simulink model "VIPR557LTStEnCtrl"  (R2024b)
settings: Solver=FixedStepDiscrete  StartTime=0.0  StopTime=10.0  FixedStep=0.01  RelTol=1e-3
undefined symbols (not defined in the file or in its folder): data, KeSMSw4SSecRwLtStLgrstUpwdDnwdOpenPos1_Val, PassStBkReclnEn_Clear, PassStBkReclnEn_Set, PassStFwdBkwdEn_Clear, PassStFwdBkwdEn_Set, SecRwRtStBkReclnEn_Clear, SecRwRtStBkReclnEn_Set, SecRwRtStFwdBkwdEn_Clear, SecRwRtStFwdBkwdEn_Set, SecRwRtStLgrstInwdOtwdEn_Clear, SecRwRtStLgrstInwdOtwdEn_Set, SecRwRtStLgrstUpwdDnwdEn_Clear, SecRwRtStLgrstUpwdDnwdEn_Set, ThdRwLtStBkReclnEn_Clear, ThdRwLtStBkReclnEn_Set, ThdRwLtStFwdBkwdEn_Clear, ThdRwLtStFwdBkwdEn_Set, ThdRwRtStBkReclnEn_Clear, ThdRwRtStBkReclnEn_Set, ThdRwRtStFwdBkwdEn_Clear, ThdRwRtStFwdBkwdEn_Set
libraries: simulink x1
settings Model: Creator=sn2xws  LastModifiedBy=sn55gm
settings Model: ModifiedHistory=|
  | 2024.7.3 V3.0.0 557模式流程V1.9
  | 2024.10.28 V3.0.1 6s不动三左
  | 2024.11.29 V3.0.2 7s信号未连接
  | 2024.12.2 V3.0.3 SecRwLtStLgrstOtwdInwdStgDone错误使用SecRwLtStLgrstUpwdDnwdStgDone信号
  | 2024.12.11 V3.0.4 CR960452
settings SolverCC: AlgebraicLoopSolver=TrustRegion
settings DataIOCC: SaveFormat=StructureWithTime  ReturnWorkspaceOutputs=off
settings OptimizationCC: DefaultParameterBehavior=Inlined  EnhancedBackFolding=on  PassReuseOutputArgsAs=Individual arguments  ZeroExternalMemoryAtStartup=off  ZeroInternalMemoryAtStartup=off  OptimizeBlockOrder=speed  DifferentSizesBufferReuse=on  OptimizationCustomize=off  EfficientTunableParamExpr=on
settings DebuggingCC: ParameterTunabilityLossMsg=error  UnconnectedInputMsg=warning  UnconnectedOutputMsg=warning  UnconnectedLineMsg=warning  ArithmeticOperatorsInVariantConditions=warning
settings ModelReferenceCC: EnableRefExpFcnMdlSchedulingChecks=on
settings SFSimCC: MATLABDynamicMemAlloc=off  CustomCodeUndefinedFunction=UseInterfaceOnly
settings RTWCC: Description=AUTOSAR  SystemTargetFile=autosar.tlc  GenCodeOnly=on  TemplateMakefile=ert_default_tmf  GenerateReport=on  IncludeHyperlinkInReport=on  LaunchReport=on  DataTypeReplacement=CDataTypesFixedWidth  GenerateTraceInfo=on  GenerateTraceReport=on  GenerateTraceReportSl=on  GenerateTraceReportSf=on  GenerateTraceReportEml=on  GPUComputeCapability=3.5
settings CodeAppCC: ForceParamTrailComments=on  IgnoreCustomStorageClasses=off  OperatorAnnotations=on  SimulinkDataObjDesc=on  SFDataObjDesc=on  InsertBlockDesc=on
settings STFCustomTargetCC: TargetLangStandard=C99 (ISO)  MultiwordLength=256  ParMdlRefBuildCompliant=on  CompOptLevelCompliant=on  IncludeMdlTerminateFcn=off  CombineOutputUpdateFcns=on  SuppressErrorStatus=on  ERTCustomFileBanners=on  SupportNonFinite=off  SupportComplex=off  SupportContinuousTime=off  SupportNonInlinedSFcns=off  RemoveResetFunc=on  MATLABClassNameForMDSCustomization=Simulink.SoftwareTarget.ERTCustomization  AutosarCompliant=on  UseToolchainInfoCompliant=on  LookupTableObjectStructAxisOrder=2,1,3,4,...  LUTObjectStructOrderEvenSpacing=Size,Table,Breakpoints  SystemTargetFile=autosar.tlc
settings ERTTargetCC: TargetLangStandard=C99 (ISO)  ConcurrentExecutionCompliant=off  IncludeMdlTerminateFcn=off  SuppressErrorStatus=on  SupportNonFinite=off  SupportComplex=off  ModelStepFunctionPrototypeControlCompliant=off  CPPClassGenCompliant=off  AutosarCompliant=on  LookupTableObjectStructAxisOrder=2,1,3,4,...  LUTObjectStructOrderEvenSpacing=Size,Table,Breakpoints  ERTCustomFileTemplate=example_file_process.tlc  ERTFilePackagingFormat=Compact  BooleanTrueId=TRUE  BooleanFalseId=FALSE  DynamicArrayContainerType=coder::array

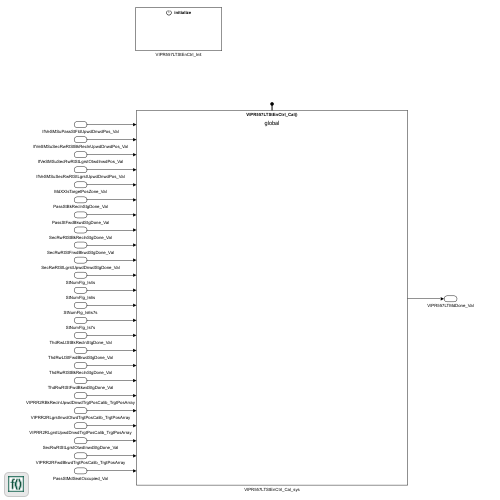
[thumbnail: Simulink's stored preview of the top-level diagram]
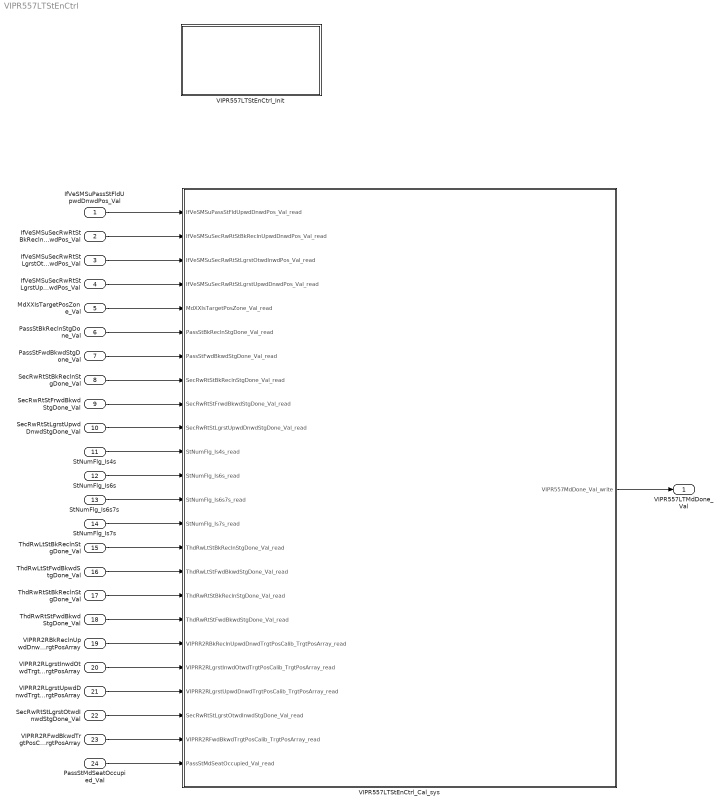
== system VIPR557LTStEnCtrl ==
  IfVeSMSuPassStFldUpwdDnwdPos_Val : Inport  OutDataTypeStr=uint16  PortDimensions=1
  IfVeSMSuSecRwRtStBkReclnUpwdDnwdPos_Val : Inport  Port=2  OutDataTypeStr=uint16  PortDimensions=1
  IfVeSMSuSecRwRtStLgrstOtwdInwdPos_Val : Inport  Port=3  OutDataTypeStr=uint16  PortDimensions=1
  IfVeSMSuSecRwRtStLgrstUpwdDnwdPos_Val : Inport  Port=4  OutDataTypeStr=uint16  PortDimensions=1
  MdXXIsTargetPosZone_Val : Inport  Port=5  OutDataTypeStr=uint32  PortDimensions=1
  PassStBkReclnStgDone_Val : Inport  Port=6  OutDataTypeStr=boolean  PortDimensions=1
  PassStFwdBkwdStgDone_Val : Inport  Port=7  OutDataTypeStr=boolean  PortDimensions=1
  SecRwRtStBkReclnStgDone_Val : Inport  Port=8  OutDataTypeStr=boolean  PortDimensions=1
  SecRwRtStFrwdBkwdStgDone_Val : Inport  Port=9  OutDataTypeStr=boolean  PortDimensions=1
  SecRwRtStLgrstUpwdDnwdStgDone_Val : Inport  Port=10  OutDataTypeStr=boolean  PortDimensions=1
  StNumFlg_Is4s : Inport  Port=11  OutDataTypeStr=boolean  PortDimensions=1
  StNumFlg_Is6s : Inport  Port=12  OutDataTypeStr=boolean  PortDimensions=1
  StNumFlg_Is6s7s : Inport  Port=13  OutDataTypeStr=boolean  PortDimensions=1
  StNumFlg_Is7s : Inport  Port=14  OutDataTypeStr=boolean  PortDimensions=1
  ThdRwLtStBkReclnStgDone_Val : Inport  Port=15  OutDataTypeStr=boolean  PortDimensions=1
  ThdRwLtStFwdBkwdStgDone_Val : Inport  Port=16  OutDataTypeStr=boolean  PortDimensions=1
  ThdRwRtStBkReclnStgDone_Val : Inport  Port=17  OutDataTypeStr=boolean  PortDimensions=1
  ThdRwRtStFwdBkwdStgDone_Val : Inport  Port=18  OutDataTypeStr=boolean  PortDimensions=1
  VIPRR2RBkReclnUpwdDnwdTrgtPosCalib_TrgtPosArray : Inport  Description=|  Port=19  OutDataTypeStr=uint16  PortDimensions=3
      | 0:Pos
      | 1:Max
      | 2:Min
  VIPRR2RLgrstInwdOtwdTrgtPosCalib_TrgtPosArray : Inport  Description=|  Port=20  OutDataTypeStr=uint16  PortDimensions=3
      | 0:Pos
      | 1:Max
      | 2:Min
  VIPRR2RLgrstUpwdDnwdTrgtPosCalib_TrgtPosArray : Inport  Description=|  Port=21  OutDataTypeStr=uint16  PortDimensions=3
      | 0:Pos
      | 1:Max
      | 2:Min
  SecRwRtStLgrstOtwdInwdStgDone_Val : Inport  Port=22  OutDataTypeStr=boolean  PortDimensions=1
  VIPRR2RFwdBkwdTrgtPosCalib_TrgtPosArray : Inport  Description=|  Port=23  OutDataTypeStr=uint16  PortDimensions=3
      | 0:Pos
      | 1:Max
      | 2:Min
  PassStMdSeatOccupied_Val : Inport  Port=24  OutDataTypeStr=boolean  PortDimensions=1
  VIPR557LTStEnCtrl_Cal_sys : Subsystem
  VIPR557LTStEnCtrl_Init : Subsystem
  VIPR557LTMdDone_Val : Outport  OutDataTypeStr=uint8  PortDimensions=1  VectorParamsAs1DForOutWhenUnconnected=off
  wires:
  IfVeSMSuPassStFldUpwdDnwdPos_Val/1 -> VIPR557LTStEnCtrl_Cal_sys/1(IfVeSMSuPassStFldUpwdDnwdPos_Val_read)
  IfVeSMSuSecRwRtStBkReclnUpwdDnwdPos_Val/1 -> VIPR557LTStEnCtrl_Cal_sys/2(IfVeSMSuSecRwRtStBkReclnUpwdDnwdPos_Val_read)
  IfVeSMSuSecRwRtStLgrstOtwdInwdPos_Val/1 -> VIPR557LTStEnCtrl_Cal_sys/3(IfVeSMSuSecRwRtStLgrstOtwdInwdPos_Val_read)
  IfVeSMSuSecRwRtStLgrstUpwdDnwdPos_Val/1 -> VIPR557LTStEnCtrl_Cal_sys/4(IfVeSMSuSecRwRtStLgrstUpwdDnwdPos_Val_read)
  MdXXIsTargetPosZone_Val/1 -> VIPR557LTStEnCtrl_Cal_sys/5(MdXXIsTargetPosZone_Val_read)
  PassStBkReclnStgDone_Val/1 -> VIPR557LTStEnCtrl_Cal_sys/6(PassStBkReclnStgDone_Val_read)
  PassStFwdBkwdStgDone_Val/1 -> VIPR557LTStEnCtrl_Cal_sys/7(PassStFwdBkwdStgDone_Val_read)
  SecRwRtStBkReclnStgDone_Val/1 -> VIPR557LTStEnCtrl_Cal_sys/8(SecRwRtStBkReclnStgDone_Val_read)
  SecRwRtStFrwdBkwdStgDone_Val/1 -> VIPR557LTStEnCtrl_Cal_sys/9(SecRwRtStFrwdBkwdStgDone_Val_read)
  SecRwRtStLgrstUpwdDnwdStgDone_Val/1 -> VIPR557LTStEnCtrl_Cal_sys/10(SecRwRtStLgrstUpwdDnwdStgDone_Val_read)
  StNumFlg_Is4s/1 -> VIPR557LTStEnCtrl_Cal_sys/11(StNumFlg_Is4s_read)
  StNumFlg_Is6s/1 -> VIPR557LTStEnCtrl_Cal_sys/12(StNumFlg_Is6s_read)
  StNumFlg_Is6s7s/1 -> VIPR557LTStEnCtrl_Cal_sys/13(StNumFlg_Is6s7s_read)
  StNumFlg_Is7s/1 -> VIPR557LTStEnCtrl_Cal_sys/14(StNumFlg_Is7s_read)
  ThdRwLtStBkReclnStgDone_Val/1 -> VIPR557LTStEnCtrl_Cal_sys/15(ThdRwLtStBkReclnStgDone_Val_read)
  ThdRwLtStFwdBkwdStgDone_Val/1 -> VIPR557LTStEnCtrl_Cal_sys/16(ThdRwLtStFwdBkwdStgDone_Val_read)
  ThdRwRtStBkReclnStgDone_Val/1 -> VIPR557LTStEnCtrl_Cal_sys/17(ThdRwRtStBkReclnStgDone_Val_read)
  ThdRwRtStFwdBkwdStgDone_Val/1 -> VIPR557LTStEnCtrl_Cal_sys/18(ThdRwRtStFwdBkwdStgDone_Val_read)
  VIPRR2RBkReclnUpwdDnwdTrgtPosCalib_TrgtPosArray/1 -> VIPR557LTStEnCtrl_Cal_sys/19(VIPRR2RBkReclnUpwdDnwdTrgtPosCalib_TrgtPosArray_read)
  VIPRR2RLgrstInwdOtwdTrgtPosCalib_TrgtPosArray/1 -> VIPR557LTStEnCtrl_Cal_sys/20(VIPRR2RLgrstInwdOtwdTrgtPosCalib_TrgtPosArray_read)
  VIPRR2RLgrstUpwdDnwdTrgtPosCalib_TrgtPosArray/1 -> VIPR557LTStEnCtrl_Cal_sys/21(VIPRR2RLgrstUpwdDnwdTrgtPosCalib_TrgtPosArray_read)
  VIPR557LTStEnCtrl_Cal_sys/1(VIPR557MdDone_Val_write) -> VIPR557LTMdDone_Val/1
  SecRwRtStLgrstOtwdInwdStgDone_Val/1 -> VIPR557LTStEnCtrl_Cal_sys/22(SecRwRtStLgrstOtwdInwdStgDone_Val_read)
  VIPRR2RFwdBkwdTrgtPosCalib_TrgtPosArray/1 -> VIPR557LTStEnCtrl_Cal_sys/23(VIPRR2RFwdBkwdTrgtPosCalib_TrgtPosArray_read)
  PassStMdSeatOccupied_Val/1 -> VIPR557LTStEnCtrl_Cal_sys/24(PassStMdSeatOccupied_Val_read)

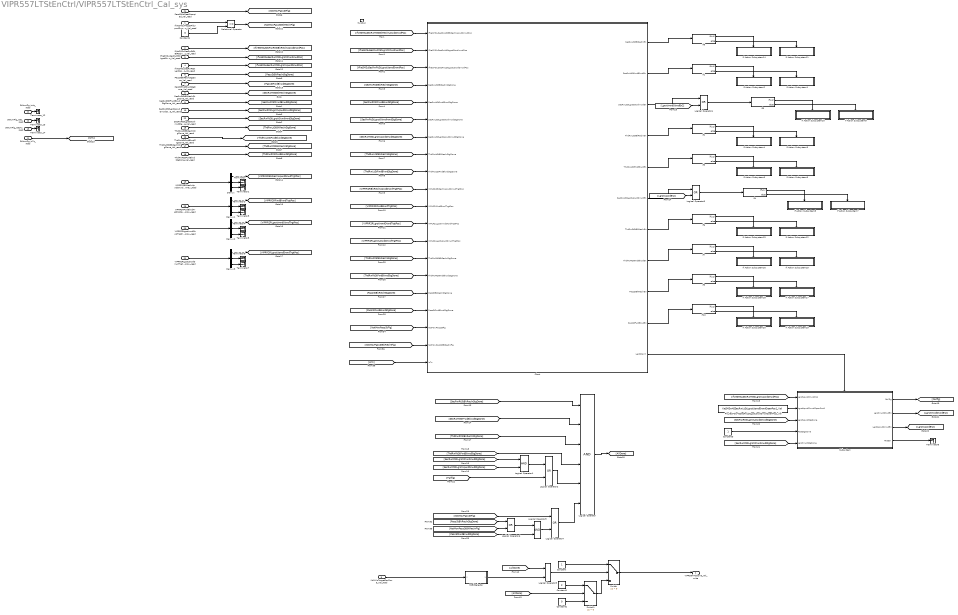
== system VIPR557LTStEnCtrl/VIPR557LTStEnCtrl_Cal_sys ==
  IfVeSMSuPassStFldUpwdDnwdPos_Val_read : Inport
  IfVeSMSuSecRwRtStBkReclnUpwdDnwdPos_Val_read : Inport  Port=2
  IfVeSMSuSecRwRtStLgrstOtwdInwdPos_Val_read : Inport  Port=3
  IfVeSMSuSecRwRtStLgrstUpwdDnwdPos_Val_read : Inport  Port=4
  MdXXIsTargetPosZone_Val_read : Inport  Port=5
  PassStBkReclnStgDone_Val_read : Inport  Port=6
  PassStFwdBkwdStgDone_Val_read : Inport  Port=7
  SecRwRtStBkReclnStgDone_Val_read : Inport  Port=8
  SecRwRtStFrwdBkwdStgDone_Val_read : Inport  Port=9
  SecRwRtStLgrstUpwdDnwdStgDone_Val_read : Inport  Port=10
  StNumFlg_Is4s_read : Inport  Port=11
  StNumFlg_Is6s_read : Inport  Port=12
  StNumFlg_Is6s7s_read : Inport  Port=13
  StNumFlg_Is7s_read : Inport  Port=14
  ThdRwLtStBkReclnStgDone_Val_read : Inport  Port=15
  ThdRwLtStFwdBkwdStgDone_Val_read : Inport  Port=16
  ThdRwRtStBkReclnStgDone_Val_read : Inport  Port=17
  ThdRwRtStFwdBkwdStgDone_Val_read : Inport  Port=18
  VIPRR2RBkReclnUpwdDnwdTrgtPosCalib_TrgtPosArray_read : Inport  Port=19
  VIPRR2RLgrstInwdOtwdTrgtPosCalib_TrgtPosArray_read : Inport  Port=20
  VIPRR2RLgrstUpwdDnwdTrgtPosCalib_TrgtPosArray_read : Inport  Port=21
  SecRwRtStLgrstOtwdInwdStgDone_Val_read : Inport  Port=22
  VIPRR2RFwdBkwdTrgtPosCalib_TrgtPosArray_read : Inport  Port=23
  PassStMdSeatOccupied_Val_read : Inport  Port=24
  function : TriggerPort  TriggerType=function-call  IsSimulinkFunction=on  FunctionName=VIPR557LTStEnCtrl_Cal  VariantControl=(inherit)
  32BitSelector : Subsystem  mask(32 Bit Selector){BitNum=11}
      mask prompts: BitNum "Select Bit Number"
      mask help: Allows selection of a particular bit (0-31) out of a packed word up to 32 bits long. Output will be true if the bit number selected via the mask parameter is equal to one.
      mask TypeOptions BitNum: 0 | 1 | 2 | 3 | 4 | 5 | 6 | 7 | 8 | 9 | 10 | 11 | 12 | 13 | 14 | 15 | 16 | 17 | 18 | 19 | 20 | 21 | 22 | 23 | 24 | 25 | 26 | 27 | 28 | 29 | 30 | 31
      mask Display:
      | text(0.5, 0.8,'BIT','horizontalAlignment','center')
      | text(0.5, 0.5,'SELECTOR','horizontalAlignment','center')
      | text(0.5, 0.2,['-- Bit ',char(get_param(gcb,'BitNum')),' --'],'horizontalAlignment','center')
  Chart : Stateflow chart  TreatAsAtomicUnit=on
  Constant : Constant  OutDataTypeStr=uint8
  Constant1 : Constant  Value=2  OutDataTypeStr=uint8
  Constant2 : Constant  Value=0  OutDataTypeStr=uint8
  Constant3 : Constant  OutDataTypeStr=boolean
  Constant4 : Constant  Value=0  OutDataTypeStr=uint16
  Demux{,1..3} (4 alike) : Demux  Outputs=3
  If Action Subsystem1 : Subsystem  TreatAsAtomicUnit=on
  If Action Subsystem10 : Subsystem  TreatAsAtomicUnit=on
  If Action Subsystem11 : Subsystem  TreatAsAtomicUnit=on
  If Action Subsystem12 : Subsystem  TreatAsAtomicUnit=on
  If Action Subsystem13 : Subsystem  TreatAsAtomicUnit=on
  If Action Subsystem14 : Subsystem  TreatAsAtomicUnit=on
  If Action Subsystem15 : Subsystem  TreatAsAtomicUnit=on
  If Action Subsystem16 : Subsystem  TreatAsAtomicUnit=on
  If Action Subsystem17 : Subsystem  TreatAsAtomicUnit=on
  If Action Subsystem18 : Subsystem  TreatAsAtomicUnit=on
  If Action Subsystem19 : Subsystem  TreatAsAtomicUnit=on
  If Action Subsystem2 : Subsystem  TreatAsAtomicUnit=on
  If Action Subsystem20 : Subsystem  TreatAsAtomicUnit=on
  If Action Subsystem3 : Subsystem  TreatAsAtomicUnit=on
  If Action Subsystem4 : Subsystem  TreatAsAtomicUnit=on
  If Action Subsystem5 : Subsystem  TreatAsAtomicUnit=on
  If Action Subsystem6 : Subsystem  TreatAsAtomicUnit=on
  If Action Subsystem7 : Subsystem  TreatAsAtomicUnit=on
  If Action Subsystem8 : Subsystem  TreatAsAtomicUnit=on
  If Action Subsystem9 : Subsystem  TreatAsAtomicUnit=on
  If{1..10} (10 alike) : If  IfExpression=u1
  Logical Operator : Logic  Inputs=6  AllPortsSameDT=off  OutDataTypeStr=boolean
  Logical Operator1 : Logic  AllPortsSameDT=off  OutDataTypeStr=boolean
  Logical Operator{2..4,6..7} (5 alike) : Logic  Operator=OR  AllPortsSameDT=off  OutDataTypeStr=boolean
  Logical Operator5 : Logic  AllPortsSameDT=off  OutDataTypeStr=boolean
  Logical Operator9 : Logic  AllPortsSameDT=off  OutDataTypeStr=boolean
  PA_KeSMSw4SSecRwLtStLgrstUpwdDnwdOpenPos1_Val : Constant  Value=KeSMSw4SSecRwLtStLgrstUpwdDnwdOpenPos1_Val
  Relational Operator : RelationalOperator  Operator=<=  OutDataTypeStr=boolean  RndMeth=Simplest  InputSameDT=off
  Subsystem : Subsystem
  Switch : Switch  Criteria=u2 > Threshold  SaturateOnIntegerOverflow=off  InputSameDT=off
  Switch1 : Switch  Criteria=u2 > Threshold  SaturateOnIntegerOverflow=off  InputSameDT=off
  Terminator{,1..8} (9 alike) : Terminator
  Terminator_12 : Terminator
  Terminator_13 : Terminator
  Terminator_14 : Terminator
  VIPR557MdDone_Val_write : Outport  VectorParamsAs1DForOutWhenUnconnected=off
      settings: EnsureOutportIsVirtual=on
  wires:
  StNumFlg_Is4s_read/1 -> Terminator_12/1
  StNumFlg_Is6s_read/1 -> Terminator_13/1
  StNumFlg_Is6s7s_read/1 -> Terminator_14/1
  StNumFlg_Is7s_read/1 -> [Is7s]
  ThdRwLtStBkReclnStgDone_Val_read/1 -> [ThdRwLtStBkReclnStgDone]
  SecRwRtStFrwdBkwdStgDone_Val_read/1 -> [SecRwRtStFrwdBkwdStgDone]
  SecRwRtStLgrstUpwdDnwdStgDone_Val_read/1 -> [SecRwRtStLgrstUpwdDnwdStgDone]
  SecRwRtStBkReclnStgDone_Val_read/1 -> [SecRwRtStBkReclnStgDone]
  ThdRwLtStFwdBkwdStgDone_Val_read/1 -> [ThdRwLtStFwdBkwdStgDone]
  SecRwRtStLgrstOtwdInwdStgDone_Val_read/1 -> [SecRwRtStLgrstOtwdInwdStgDone]
  IfVeSMSuSecRwRtStBkReclnUpwdDnwdPos_Val_read/1 -> [IfVeSMSuSecRwRtStBkReclnUpwdDnwdPos]
  IfVeSMSuSecRwRtStLgrstOtwdInwdPos_Val_read/1 -> [IfVeSMSuSecRwRtStLgrstOtwdInwdPos]
  IfVeSMSuSecRwRtStLgrstUpwdDnwdPos_Val_read/1 -> [IfVeSMSuSecRwRtStLgrstUpwdDnwdPos]
  ThdRwRtStBkReclnStgDone_Val_read/1 -> [ThdRwRtStBkReclnStgDone]
  ThdRwRtStFwdBkwdStgDone_Val_read/1 -> [ThdRwRtStFwdBkwdStgDone]
  PassStBkReclnStgDone_Val_read/1 -> [PassStBkReclnStgDone]
  PassStFwdBkwdStgDone_Val_read/1 -> [PassStFwdBkwdStgDone]
  Demux2/1 -> [VIPRR2RLgrstInwdOtwdTrgtPos]
  VIPRR2RBkReclnUpwdDnwdTrgtPosCalib_TrgtPosArray_read/1 -> Demux/1
  VIPRR2RFwdBkwdTrgtPosCalib_TrgtPosArray_read/1 -> Demux1/1
  VIPRR2RLgrstUpwdDnwdTrgtPosCalib_TrgtPosArray_read/1 -> Demux3/1
  Demux3/1 -> [VIPRR2RLgrstUpwdDnwdTrgtPos]
  Demux3/2 -> Terminator6/1
  Demux1/3 -> Terminator3/1
  Demux/3 -> Terminator1/1
  Demux3/3 -> Terminator7/1
  Demux/1 -> [VIPRR2RBkReclnUpwdDnwdTrgtPos]
  Demux1/1 -> [VIPRR2RFwdBkwdTrgtPos]
  Demux2/2 -> Terminator4/1
  VIPRR2RLgrstInwdOtwdTrgtPosCalib_TrgtPosArray_read/1 -> Demux2/1
  Demux/2 -> Terminator/1
  Demux2/3 -> Terminator5/1
  Demux1/2 -> Terminator2/1
  [IfVeSMSuSecRwRtStLgrstUpwdDnwdPos] -> Chart/3(IfVeSMSuSecRwLtStLgrstUpwdDnwdPos)
  [SecRwRtStFrwdBkwdStgDone] -> Logical Operator/2
  Logical Operator4/1 -> If5/1
  Chart/11(LgrstOpn()) -> Subsystem/Trigger
  [LgrstUpwdEn2] -> Logical Operator3/2
  Chart/3(SecRwLtStLgrstOtwdInwdEn) -> Logical Operator4/1
  Chart/5(ThdRwLtStFwdBkwdEn) -> If3/1
  If5/2 -> If Action Subsystem9/Action
  [SecRwRtStLgrstOtwdInwdStgDone] -> Logical Operator1/1
  If4/1 -> If Action Subsystem8/Action
  Logical Operator2/1 -> Logical Operator/5
  [LgrstInwdOtwdEn2] -> Logical Operator4/2
  Chart/6(SecRwLtStLgrstUpwdDnwdEn) -> Logical Operator3/1
  Chart/4(ThdRwLtStBkReclnEn) -> If2/1
  If1/1 -> If Action Subsystem2/Action
  [IfVeSMSuSecRwRtStLgrstOtwdInwdPos] -> Chart/2(IfVeSMSuSecRwLtStLgrstOtwdInwdPos)
  Subsystem/2(LgrstInwdOtwdEn) -> [LgrstInwdOtwdEn2]
  Logical Operator/1 -> [AllDone]
  [VIPRR2RLgrstInwdOtwdTrgtPos] -> Chart/12(VIPLR2LLgrstInwdOtwdTrgtPos)
  If1/2 -> If Action Subsystem1/Action
  If4/2 -> If Action Subsystem7/Action
  Subsystem/1(Failflg) -> [Failflg]
  [SecRwRtStBkReclnStgDone] -> Logical Operator/1
  Subsystem/4(FtrstEn) -> Terminator8/1
  If8/2 -> If Action Subsystem11/Action
  If2/2 -> If Action Subsystem3/Action
  If3/1 -> If Action Subsystem6/Action
  [SecRwRtStLgrstUpwdDnwdStgDone] -> Subsystem/3(LgrstUpwdStgDone)
  Chart/1(SecRwLtStBkReclnEn) -> If8/1
  [ThdRwRtStFwdBkwdStgDone] -> Logical Operator/4
  [SecRwRtStLgrstUpwdDnwdStgDone] -> Logical Operator1/2
  [Failflg] -> Logical Operator2/2
  [SecRwRtStLgrstOtwdInwdStgDone] -> Subsystem/5(LgrstInwdStgDone)
  [SecRwRtStLgrstUpwdDnwdStgDone] -> Chart/7(SecRwLtStLgrstUpwdDnwdStgDone)
  Subsystem/3(LgrstUpwdDnwdEn) -> [LgrstUpwdEn2]
  Constant3/1 -> Subsystem/4(FtrstStgDone)
  If5/1 -> If Action Subsystem10/Action
  [SecRwRtStFrwdBkwdStgDone] -> Chart/5(SecRwLtStFrwdBkwdStgDone)
  If8/1 -> If Action Subsystem14/Action
  [VIPRR2RLgrstUpwdDnwdTrgtPos] -> Chart/13(VIPLR2LLgrstUpwdDnwdTrgtPos)
  [VIPRR2RFwdBkwdTrgtPos] -> Chart/11(VIPLR2LFwdBkwdTrgtPos)
  Chart/2(SecRwLtStFrwdBkwdEn) -> If1/1
  Logical Operator1/1 -> Logical Operator2/1
  [SecRwRtStBkReclnStgDone] -> Chart/4(SecRwLtStBkReclnStgDone)
  [SecRwRtStLgrstOtwdInwdStgDone] -> Chart/6(SecRwLtStLgrstOtwdInwdStgDone)
  If3/2 -> If Action Subsystem5/Action
  If2/1 -> If Action Subsystem4/Action
  [ThdRwLtStBkReclnStgDone] -> Chart/8(ThdRwLtStBkReclnStgDone)
  PA_KeSMSw4SSecRwLtStLgrstUpwdDnwdOpenPos1_Val/1 -> Subsystem/2(LgrstUpwdDnwdOpenPos1)
  [IfVeSMSuSecRwRtStBkReclnUpwdDnwdPos] -> Chart/1(IfVeSMSuSecRwLtStBkReclnUpwdDnwdPos)
  Logical Operator3/1 -> If4/1
  [VIPRR2RBkReclnUpwdDnwdTrgtPos] -> Chart/10(VIPLR2LBkReclnUpwdDnwdTrgtPos)
  [ThdRwLtStFwdBkwdStgDone] -> Chart/9(ThdRwLtStFwdBkwdStgDone)
  [ThdRwRtStBkReclnStgDone] -> Logical Operator/3
  [IfVeSMSuSecRwRtStLgrstUpwdDnwdPos] -> Subsystem/1(LgrstUpwdDnwdPos)
  [AllDone] -> Logical Operator9/1
  Constant2/1 -> Switch1/3
  32BitSelector/1(y) -> Logical Operator9/2
  Constant1/1 -> Switch1/1
  Switch1/1 -> Switch/3
  Logical Operator9/1 -> Switch/2
  Constant/1 -> Switch/1
  [AllDone] -> Switch1/2
  MdXXIsTargetPosZone_Val_read/1 -> 32BitSelector/1(x)
  Switch/1 -> VIPR557MdDone_Val_write/1
  [PassStBkReclnStgDone] -> Chart/16(PassStBkReclnStgDone)
  Logical Operator7/1 -> Logical Operator/6
  Logical Operator5/1 -> Logical Operator7/2
  IfVeSMSuPassStFldUpwdDnwdPos_Val_read/1 -> Relational Operator/1
  Constant4/1 -> Relational Operator/2
  PassStMdSeatOccupied_Val_read/1 -> [NotMovPassStFlg]
  [NotMovPassStFlg] -> Logical Operator7/1
  Relational Operator/1 -> [NotMovPassStBkReclnFlg]
  [PassStBkReclnStgDone] -> Logical Operator6/1
  [NotMovPassStBkReclnFlg] -> Logical Operator6/2
  Logical Operator6/1 -> Logical Operator5/1
  [PassStFwdBkwdStgDone] -> Logical Operator5/2
  [ThdRwRtStBkReclnStgDone] -> Chart/14(ThdRwRtStBkReclnStgDone)
  [ThdRwRtStFwdBkwdStgDone] -> Chart/15(ThdRwRtStFwdBkwdStgDone)
  [NotMovPassStFlg] -> Chart/18(NotMovPassStFlg)
  [PassStFwdBkwdStgDone] -> Chart/17(PassStFwdBkwdStgDone)
  [NotMovPassStBkReclnFlg] -> Chart/19(NotMovPassStBkReclnFlg)
  If6/2 -> If Action Subsystem12/Action
  If6/1 -> If Action Subsystem13/Action
  Chart/7(ThdRwRtStBkReclnEn) -> If6/1
  Chart/8(ThdRwRtStFwdBkwdEn) -> If7/1
  If7/1 -> If Action Subsystem16/Action
  If7/2 -> If Action Subsystem15/Action
  If9/2 -> If Action Subsystem17/Action
  If9/1 -> If Action Subsystem18/Action
  Chart/9(PassStBkReclnEn) -> If9/1
  Chart/10(PassStFwdBkwdEn) -> If10/1
  If10/1 -> If Action Subsystem20/Action
  If10/2 -> If Action Subsystem19/Action
  [Is7s] -> Chart/20(is7s)

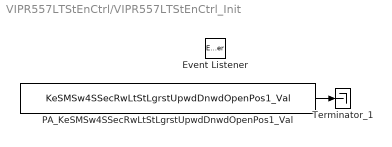
== system VIPR557LTStEnCtrl/VIPR557LTStEnCtrl_Init ==
  Event Listener : EventListener  EventName=reset
  PA_KeSMSw4SSecRwLtStLgrstUpwdDnwdOpenPos1_Val : Constant  Value=KeSMSw4SSecRwLtStLgrstUpwdDnwdOpenPos1_Val
  Terminator_1 : Terminator
  wires:
  PA_KeSMSw4SSecRwLtStLgrstUpwdDnwdOpenPos1_Val/1 -> Terminator_1/1

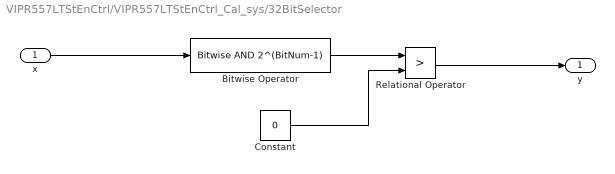
== system VIPR557LTStEnCtrl/VIPR557LTStEnCtrl_Cal_sys/32BitSelector ==
  x : Inport
  Bitwise Operator : simulink/Logic and Bit Operations/Bitwise Operator  logicop=AND  UseBitMask=on  BitMask=2^(BitNum-1)  BitMaskRealWorld=Stored Integer
  Constant : Constant  Value=0  OutDataTypeStr=uint32
  Relational Operator : RelationalOperator  Operator=>  OutDataTypeStr=boolean  RndMeth=Simplest  InputSameDT=off
  y : Outport  VectorParamsAs1DForOutWhenUnconnected=off
  wires:
  Relational Operator/1 -> y/1
  Constant/1 -> Relational Operator/2
  x/1 -> Bitwise Operator/1
  Bitwise Operator/1 -> Relational Operator/1

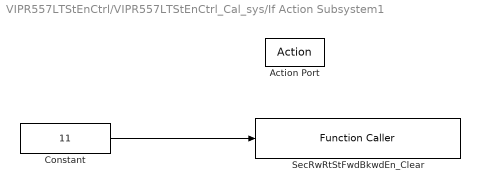
== system VIPR557LTStEnCtrl/VIPR557LTStEnCtrl_Cal_sys/If Action Subsystem1 ==
  Action Port : ActionPort  ActionPortLabel=else
  Constant : Constant  Value=11  OutDataTypeStr=uint8
  SecRwRtStFwdBkwdEn_Clear : FunctionCaller  FunctionPrototype=SecRwRtStFwdBkwdEn_Clear(data)  InputArgumentSpecifications=uint8(1)  OutputArgumentSpecifications=<Enter example>
  wires:
  Constant/1 -> SecRwRtStFwdBkwdEn_Clear/1

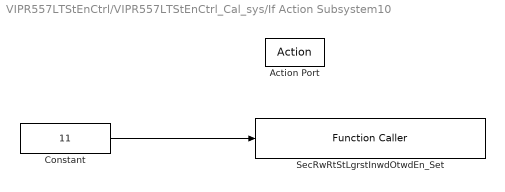
== system VIPR557LTStEnCtrl/VIPR557LTStEnCtrl_Cal_sys/If Action Subsystem10 ==
  Action Port : ActionPort  ActionPortLabel=if(u1)
  Constant : Constant  Value=11  OutDataTypeStr=uint8
  SecRwRtStLgrstInwdOtwdEn_Set : FunctionCaller  FunctionPrototype=SecRwRtStLgrstInwdOtwdEn_Set(data)  InputArgumentSpecifications=uint8(1)  OutputArgumentSpecifications=<Enter example>
  wires:
  Constant/1 -> SecRwRtStLgrstInwdOtwdEn_Set/1

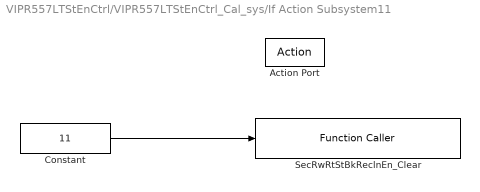
== system VIPR557LTStEnCtrl/VIPR557LTStEnCtrl_Cal_sys/If Action Subsystem11 ==
  Action Port : ActionPort  ActionPortLabel=else
  Constant : Constant  Value=11  OutDataTypeStr=uint8
  SecRwRtStBkReclnEn_Clear : FunctionCaller  FunctionPrototype=SecRwRtStBkReclnEn_Clear(data)  InputArgumentSpecifications=uint8(1)  OutputArgumentSpecifications=<Enter example>
  wires:
  Constant/1 -> SecRwRtStBkReclnEn_Clear/1

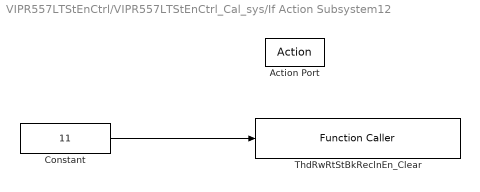
== system VIPR557LTStEnCtrl/VIPR557LTStEnCtrl_Cal_sys/If Action Subsystem12 ==
  Action Port : ActionPort  ActionPortLabel=else
  Constant : Constant  Value=11  OutDataTypeStr=uint8
  ThdRwRtStBkReclnEn_Clear : FunctionCaller  FunctionPrototype=ThdRwRtStBkReclnEn_Clear(data)  InputArgumentSpecifications=uint8(1)  OutputArgumentSpecifications=<Enter example>
  wires:
  Constant/1 -> ThdRwRtStBkReclnEn_Clear/1

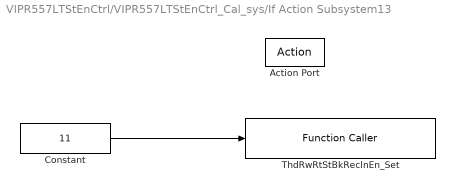
== system VIPR557LTStEnCtrl/VIPR557LTStEnCtrl_Cal_sys/If Action Subsystem13 ==
  Action Port : ActionPort  ActionPortLabel=if(u1)
  Constant : Constant  Value=11  OutDataTypeStr=uint8
  ThdRwRtStBkReclnEn_Set : FunctionCaller  FunctionPrototype=ThdRwRtStBkReclnEn_Set(data)  InputArgumentSpecifications=uint8(1)  OutputArgumentSpecifications=<Enter example>
  wires:
  Constant/1 -> ThdRwRtStBkReclnEn_Set/1

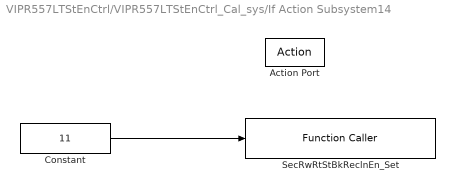
== system VIPR557LTStEnCtrl/VIPR557LTStEnCtrl_Cal_sys/If Action Subsystem14 ==
  Action Port : ActionPort  ActionPortLabel=if(u1)
  Constant : Constant  Value=11  OutDataTypeStr=uint8
  SecRwRtStBkReclnEn_Set : FunctionCaller  FunctionPrototype=SecRwRtStBkReclnEn_Set(data)  InputArgumentSpecifications=uint8(1)  OutputArgumentSpecifications=<Enter example>
  wires:
  Constant/1 -> SecRwRtStBkReclnEn_Set/1

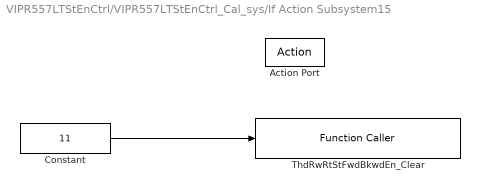
== system VIPR557LTStEnCtrl/VIPR557LTStEnCtrl_Cal_sys/If Action Subsystem15 ==
  Action Port : ActionPort  ActionPortLabel=else
  Constant : Constant  Value=11  OutDataTypeStr=uint8
  ThdRwRtStFwdBkwdEn_Clear : FunctionCaller  FunctionPrototype=ThdRwRtStFwdBkwdEn_Clear(data)  InputArgumentSpecifications=uint8(1)  OutputArgumentSpecifications=<Enter example>
  wires:
  Constant/1 -> ThdRwRtStFwdBkwdEn_Clear/1

== system VIPR557LTStEnCtrl/VIPR557LTStEnCtrl_Cal_sys/If Action Subsystem16 ==
  Action Port : ActionPort  ActionPortLabel=if(u1)
  Constant : Constant  Value=11  OutDataTypeStr=uint8
  ThdRwRtStFwdBkwdEn_Set : FunctionCaller  FunctionPrototype=ThdRwRtStFwdBkwdEn_Set(data)  InputArgumentSpecifications=uint8(1)  OutputArgumentSpecifications=<Enter example>
  wires:
  Constant/1 -> ThdRwRtStFwdBkwdEn_Set/1

== system VIPR557LTStEnCtrl/VIPR557LTStEnCtrl_Cal_sys/If Action Subsystem17 ==
  Action Port : ActionPort  ActionPortLabel=else
  Constant : Constant  Value=11  OutDataTypeStr=uint8
  PassStBkReclnEn_Clear : FunctionCaller  FunctionPrototype=PassStBkReclnEn_Clear(data)  InputArgumentSpecifications=uint8(1)  OutputArgumentSpecifications=<Enter example>
  wires:
  Constant/1 -> PassStBkReclnEn_Clear/1

== system VIPR557LTStEnCtrl/VIPR557LTStEnCtrl_Cal_sys/If Action Subsystem18 ==
  Action Port : ActionPort  ActionPortLabel=if(u1)
  Constant : Constant  Value=11  OutDataTypeStr=uint8
  PassStBkReclnEn_Set : FunctionCaller  FunctionPrototype=PassStBkReclnEn_Set(data)  InputArgumentSpecifications=uint8(1)  OutputArgumentSpecifications=<Enter example>
  wires:
  Constant/1 -> PassStBkReclnEn_Set/1

== system VIPR557LTStEnCtrl/VIPR557LTStEnCtrl_Cal_sys/If Action Subsystem19 ==
  Action Port : ActionPort  ActionPortLabel=else
  Constant : Constant  Value=11  OutDataTypeStr=uint8
  PassStFwdBkwdEn_Clear : FunctionCaller  FunctionPrototype=PassStFwdBkwdEn_Clear(data)  InputArgumentSpecifications=uint8(1)  OutputArgumentSpecifications=<Enter example>
  wires:
  Constant/1 -> PassStFwdBkwdEn_Clear/1

== system VIPR557LTStEnCtrl/VIPR557LTStEnCtrl_Cal_sys/If Action Subsystem2 ==
  Action Port : ActionPort  ActionPortLabel=if(u1)
  Constant : Constant  Value=11  OutDataTypeStr=uint8
  SecRwRtStFwdBkwdEn_Set : FunctionCaller  FunctionPrototype=SecRwRtStFwdBkwdEn_Set(data)  InputArgumentSpecifications=uint8(1)  OutputArgumentSpecifications=<Enter example>
  wires:
  Constant/1 -> SecRwRtStFwdBkwdEn_Set/1

== system VIPR557LTStEnCtrl/VIPR557LTStEnCtrl_Cal_sys/If Action Subsystem20 ==
  Action Port : ActionPort  ActionPortLabel=if(u1)
  Constant : Constant  Value=11  OutDataTypeStr=uint8
  PassStFwdBkwdEn_Set : FunctionCaller  FunctionPrototype=PassStFwdBkwdEn_Set(data)  InputArgumentSpecifications=uint8(1)  OutputArgumentSpecifications=<Enter example>
  wires:
  Constant/1 -> PassStFwdBkwdEn_Set/1

== system VIPR557LTStEnCtrl/VIPR557LTStEnCtrl_Cal_sys/If Action Subsystem3 ==
  note: Delete block
  note: Delete block
  Action Port : ActionPort  ActionPortLabel=else
  Constant : Constant  Value=11  OutDataTypeStr=uint8
  ThdRwLtStBkReclnEn_Clear : FunctionCaller  FunctionPrototype=ThdRwLtStBkReclnEn_Clear(data)  InputArgumentSpecifications=uint8(1)  OutputArgumentSpecifications=<Enter example>
  wires:
  Constant/1 -> ThdRwLtStBkReclnEn_Clear/1

== system VIPR557LTStEnCtrl/VIPR557LTStEnCtrl_Cal_sys/If Action Subsystem4 ==
  note: Delete block
  note: Delete block
  Action Port : ActionPort  ActionPortLabel=if(u1)
  Constant : Constant  Value=11  OutDataTypeStr=uint8
  ThdRwLtStBkReclnEn_Set : FunctionCaller  FunctionPrototype=ThdRwLtStBkReclnEn_Set(data)  InputArgumentSpecifications=uint8(1)  OutputArgumentSpecifications=<Enter example>
  wires:
  Constant/1 -> ThdRwLtStBkReclnEn_Set/1

== system VIPR557LTStEnCtrl/VIPR557LTStEnCtrl_Cal_sys/If Action Subsystem5 ==
  note: Delete block
  note: Delete block
  Action Port : ActionPort  ActionPortLabel=else
  Constant : Constant  Value=11  OutDataTypeStr=uint8
  ThdRwLtStFwdBkwdEn_Clear : FunctionCaller  FunctionPrototype=ThdRwLtStFwdBkwdEn_Clear(data)  InputArgumentSpecifications=uint8(1)  OutputArgumentSpecifications=<Enter example>
  wires:
  Constant/1 -> ThdRwLtStFwdBkwdEn_Clear/1

== system VIPR557LTStEnCtrl/VIPR557LTStEnCtrl_Cal_sys/If Action Subsystem6 ==
  note: Delete block
  note: Delete block
  Action Port : ActionPort  ActionPortLabel=if(u1)
  Constant : Constant  Value=11  OutDataTypeStr=uint8
  ThdRwLtStFwdBkwdEn_Set : FunctionCaller  FunctionPrototype=ThdRwLtStFwdBkwdEn_Set(data)  InputArgumentSpecifications=uint8(1)  OutputArgumentSpecifications=<Enter example>
  wires:
  Constant/1 -> ThdRwLtStFwdBkwdEn_Set/1

== system VIPR557LTStEnCtrl/VIPR557LTStEnCtrl_Cal_sys/If Action Subsystem7 ==
  Action Port : ActionPort  ActionPortLabel=else
  Constant : Constant  Value=11  OutDataTypeStr=uint8
  SecRwRtStLgrstUpwdDnwdEn_Clear : FunctionCaller  FunctionPrototype=SecRwRtStLgrstUpwdDnwdEn_Clear(data)  InputArgumentSpecifications=uint8(1)  OutputArgumentSpecifications=<Enter example>
  wires:
  Constant/1 -> SecRwRtStLgrstUpwdDnwdEn_Clear/1

== system VIPR557LTStEnCtrl/VIPR557LTStEnCtrl_Cal_sys/If Action Subsystem8 ==
  Action Port : ActionPort  ActionPortLabel=if(u1)
  Constant : Constant  Value=11  OutDataTypeStr=uint8
  SecRwRtStLgrstUpwdDnwdEn_Set : FunctionCaller  FunctionPrototype=SecRwRtStLgrstUpwdDnwdEn_Set(data)  InputArgumentSpecifications=uint8(1)  OutputArgumentSpecifications=<Enter example>
  wires:
  Constant/1 -> SecRwRtStLgrstUpwdDnwdEn_Set/1

== system VIPR557LTStEnCtrl/VIPR557LTStEnCtrl_Cal_sys/If Action Subsystem9 ==
  Action Port : ActionPort  ActionPortLabel=else
  Constant : Constant  Value=11  OutDataTypeStr=uint8
  SecRwRtStLgrstInwdOtwdEn_Clear : FunctionCaller  FunctionPrototype=SecRwRtStLgrstInwdOtwdEn_Clear(data)  InputArgumentSpecifications=uint8(1)  OutputArgumentSpecifications=<Enter example>
  wires:
  Constant/1 -> SecRwRtStLgrstInwdOtwdEn_Clear/1

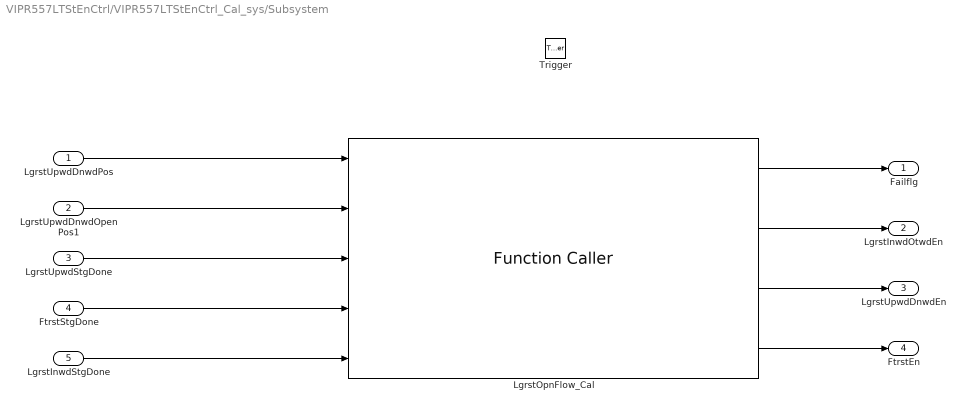
== system VIPR557LTStEnCtrl/VIPR557LTStEnCtrl_Cal_sys/Subsystem ==
  LgrstUpwdDnwdPos : Inport
  LgrstUpwdDnwdOpenPos1 : Inport  Port=2
  LgrstUpwdStgDone : Inport  Port=3
  FtrstStgDone : Inport  Port=4
  LgrstInwdStgDone : Inport  Port=5
  Trigger : TriggerPort  TriggerType=function-call  VariantControl=Variant  PortDimensions=1
  LgrstOpnFlow_Cal : FunctionCaller  FunctionPrototype=[Failflg,LgrstInwdOtwdEn,LgrstUpwdDnwdEn,FtrstEn] = LgrstOpnFlow_Cal(LgrstUpwdDnwdPos,LgrstUpwdDnwdOpenPos1,LgrstUpwdStgDone,FtrstStgDone,LgrstInwdStgDone)  InputArgumentSpecifications=uint16(1), uint16(1), boolean(true), boolean(true), boolean(true)  OutputArgumentSpecifications=boolean(true), boolean(true), boolean(true), boolean(true)
  Failflg : Outport  VectorParamsAs1DForOutWhenUnconnected=off
  LgrstInwdOtwdEn : Outport  Port=2  VectorParamsAs1DForOutWhenUnconnected=off
  LgrstUpwdDnwdEn : Outport  Port=3  VectorParamsAs1DForOutWhenUnconnected=off
  FtrstEn : Outport  Port=4  VectorParamsAs1DForOutWhenUnconnected=off
  wires:
  LgrstOpnFlow_Cal/2 -> LgrstInwdOtwdEn/1
  LgrstUpwdDnwdPos/1 -> LgrstOpnFlow_Cal/1
  LgrstOpnFlow_Cal/3 -> LgrstUpwdDnwdEn/1
  FtrstStgDone/1 -> LgrstOpnFlow_Cal/4
  LgrstUpwdStgDone/1 -> LgrstOpnFlow_Cal/3
  LgrstOpnFlow_Cal/4 -> FtrstEn/1
  LgrstInwdStgDone/1 -> LgrstOpnFlow_Cal/5
  LgrstUpwdDnwdOpenPos1/1 -> LgrstOpnFlow_Cal/2
  LgrstOpnFlow_Cal/1 -> Failflg/1

== stateflow chart VIPR557LTStEnCtrl/VIPR557LTStEnCtrl_Cal_sys/Chart ==
  (default) -> (junction 1) : {
      | ThdRwLtStBkReclnEn = 0;
      | SecRwLtStBkReclnEn = 0;
      | SecRwLtStFrwdBkwdEn = 0;
      | SecRwLtStLgrstOtwdInwdEn = 0;
      | SecRwLtStLgrstUpwdDnwdEn = 0;
      | ThdRwLtStFwdBkwdEn = 0;
      | ThdRwRtStBkReclnEn = 0;
      | ThdRwRtStFwdBkwdEn = 0;
      | PassStBkReclnEn = 0;
      | PassStFwdBkwdEn = 0;
      | }
  (junction 1) -> (junction 22) [order 1] : [!ThdRwLtStBkReclnStgDone]
  (junction 1) -> (junction 173) [order 2]
  (junction 22) -> (junction 24) : {ThdRwLtStBkReclnEn = 1;}
  (junction 173) -> (junction 175) [order 1] : [!ThdRwLtStFwdBkwdStgDone]
  (junction 175) -> (junction 169) : {ThdRwLtStFwdBkwdEn = 1;}
  (junction 173) -> (junction 26) [order 2]
  (junction 169) -> (junction 26)
  (junction 24) -> (junction 169)
  (junction 26) -> (junction 124)
  (junction 124) -> (junction 126) [order 1] : [NotMovPassStFlg]
  (junction 124) -> (junction 134) [order 2]
  (junction 126) -> (junction 129)
  (junction 134) -> (junction 136) [order 1] : [NotMovPassStBkReclnFlg ||PassStBkReclnStgDone]
  (junction 134) -> (junction 131) [order 2] : {PassStBkReclnEn =1;}
  (junction 136) -> (junction 138)
  (junction 138) -> (junction 131)
  (junction 131) -> (junction 149)
  (junction 149) -> (junction 151) [order 1] : [PassStFwdBkwdStgDone]
  (junction 149) -> (junction 155) [order 2] : {PassStFwdBkwdEn = 1;}
  (junction 151) -> (junction 153)
  (junction 153) -> (junction 155)
  (junction 129) -> (junction 153)
  (junction 155) -> (junction 38)
  (junction 38) -> (junction 40) [order 1] : [IfVeSMSuSecRwLtStBkReclnUpwdDnwdPos>VIPLR2LBkReclnUpwdDnwdTrgtPos&&!SecRwLtStBkReclnStgDone]
  (junction 38) -> (junction 44) [order 2]
  (junction 40) -> (junction 42) : {SecRwLtStBkReclnEn = 1;}
  (junction 42) -> (junction 44)
  (junction 44) -> (junction 47)
  (junction 47) -> (junction 49) [order 1] : [IfVeSMSuSecRwLtStLgrstOtwdInwdPos >VIPLR2LLgrstInwdOtwdTrgtPos &&!SecRwLtStLgrstUpwdDnwdStgDone]
  (junction 47) -> (junction 53) [order 2]
  (junction 49) -> (junction 51) : {SecRwLtStLgrstOtwdInwdEn = 1;}
  (junction 51) -> (junction 53)
  (junction 53) -> (junction 56)
  (junction 56) -> (junction 58) [order 1] : [IfVeSMSuSecRwLtStLgrstUpwdDnwdPos >VIPLR2LLgrstUpwdDnwdTrgtPos && !SecRwLtStLgrstUpwdDnwdStgDone]
  (junction 56) -> (junction 62) [order 2]
  (junction 58) -> (junction 60) : {SecRwLtStLgrstUpwdDnwdEn = 1;}
  (junction 60) -> (junction 62)
  (junction 62) -> (junction 65)
  (junction 65) -> (junction 67) [order 1] : [(IfVeSMSuSecRwLtStBkReclnUpwdDnwdPos<=VIPLR2LBkReclnUpwdDnwdTrgtPos||SecRwLtStBkReclnStgDone)&&...
      | (IfVeSMSuSecRwLtStLgrstOtwdInwdPos <=VIPLR2LLgrstInwdOtwdTrgtPos ||SecRwLtStLgrstOtwdInwdStgDone) &&...
      | (IfVeSMSuSecRwLtStLgrstUpwdDnwdPos <=VIPLR2LLgrstUpwdDnwdTrgtPos ||SecRwLtStLgrstUpwdDnwdStgDone)]
  (junction 67) -> (junction 69) [order 1] : [SecRwLtStFrwdBkwdStgDone]
  (junction 69) -> (junction 76) [order 1] : [SecRwLtStBkReclnStgDone]
  (junction 65) -> (junction 87) [order 2]
  (junction 67) -> (junction 73) [order 2] : {SecRwLtStFrwdBkwdEn =1;}
  (junction 69) -> (junction 71) [order 2] : {SecRwLtStBkReclnEn = 1;}
  (junction 76) -> (junction 78)
  (junction 78) -> (junction 71)
  (junction 71) -> (junction 81) : {LgrstOpn;}
  (junction 73) -> (junction 87)
  (junction 81) -> (junction 73)
  data: IfVeSMSuSecRwLtStBkReclnUpwdDnwdPos input; IfVeSMSuSecRwLtStLgrstOtwdInwdPos input; IfVeSMSuSecRwLtStLgrstUpwdDnwdPos input; SecRwLtStBkReclnStgDone input; SecRwLtStFrwdBkwdStgDone input; SecRwLtStLgrstOtwdInwdStgDone input; SecRwLtStLgrstUpwdDnwdStgDone input; ThdRwLtStBkReclnStgDone input; ThdRwLtStFwdBkwdStgDone input; VIPLR2LBkReclnUpwdDnwdTrgtPos input; VIPLR2LFwdBkwdTrgtPos input; VIPLR2LLgrstInwdOtwdTrgtPos input; VIPLR2LLgrstUpwdDnwdTrgtPos input; SecRwLtStBkReclnEn output boolean; SecRwLtStFrwdBkwdEn output boolean; SecRwLtStLgrstOtwdInwdEn output boolean; ThdRwLtStBkReclnEn output boolean; ThdRwLtStFwdBkwdEn output boolean; SecRwLtStLgrstUpwdDnwdEn output boolean; ThdRwRtStBkReclnEn output boolean; ThdRwRtStFwdBkwdEn output boolean; PassStBkReclnEn output boolean; PassStFwdBkwdEn output boolean; ThdRwRtStBkReclnStgDone input; ThdRwRtStFwdBkwdStgDone input; PassStBkReclnStgDone input; PassStFwdBkwdStgDone input; NotMovPassStFlg input boolean; NotMovPassStBkReclnFlg input boolean; is7s input
  events: LgrstOpn output FUNCTION_CALL_EVENT
